simulink model "led_model"  (R2020a)
settings: Solver=FixedStepAuto  StartTime=0.0  StopTime=10.0  FixedStep=1e-3  RelTol=1e-3  EnableMultiTasking=on
undefined symbols (not defined in the file): D0, D1, D10, D11, D12, D13, D2, D3, D4, D5, D6, D7, D8, D9, PTA0, PTA1, PTA2, PTB23, PTB9, PTC16, PTC17, PTC2, PTC3, PTC4, PTD0, PTD1, PTD2, PTD3
libraries: frdmk64flib x17
settings Model: ExtModeTrigDuration=5  Creator=user  LastModifiedBy=user
settings OptimizationCC: EnhancedBackFolding=on  PassReuseOutputArgsAs=Individual arguments  ZeroExternalMemoryAtStartup=off  ZeroInternalMemoryAtStartup=off  MaxStackSize=64  OptimizeBlockOrder=speed  DifferentSizesBufferReuse=on  OptimizationCustomize=off  EfficientTunableParamExpr=on
settings DebuggingCC: ParameterTunabilityLossMsg=error
settings HardwareCC: ProdBitPerPointer=32  ProdBitPerSizeT=32  ProdBitPerPtrDiffT=32  ProdLargestAtomicInteger=Long  ProdLargestAtomicFloat=Double  ProdWordSize=32  ProdHWDeviceType=ARM Compatible->ARM Cortex
settings SFSimCC: MATLABDynamicMemAlloc=off
settings RTWCC: SystemTargetFile=ert.tlc  HardwareBoard=NXP FRDM-K64F  TemplateMakefile=ert_default_tmf  Toolchain=GNU Tools for ARM Embedded Processors
settings CodeAppCC: ForceParamTrailComments=on  IgnoreCustomStorageClasses=off  OperatorAnnotations=on  SimulinkDataObjDesc=on  SFDataObjDesc=on  InsertBlockDesc=on

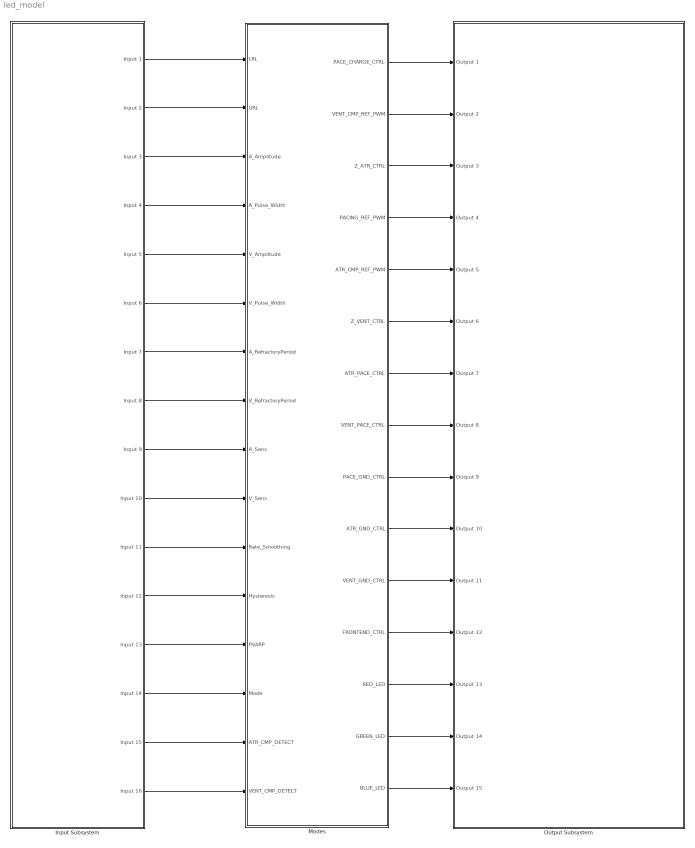
== system led_model ==
  Input Subsystem : Subsystem
  Modes : Stateflow chart  TreatAsAtomicUnit=on
  Output Subsystem : Subsystem
  wires:
  Modes/1(PACE_CHARGE_CTRL) -> Output Subsystem/1(Output 1)
  Modes/2(VENT_CMP_REF_PWM) -> Output Subsystem/2(Output 2)
  Modes/3(Z_ATR_CTRL) -> Output Subsystem/3(Output 3)
  Modes/4(PACING_REF_PWM) -> Output Subsystem/4(Output 4)
  Modes/5(ATR_CMP_REF_PWM) -> Output Subsystem/5(Output 5)
  Modes/6(Z_VENT_CTRL) -> Output Subsystem/6(Output 6)
  Modes/7(ATR_PACE_CTRL) -> Output Subsystem/7(Output 7)
  Modes/8(VENT_PACE_CTRL) -> Output Subsystem/8(Output 8)
  Modes/9(PACE_GND_CTRL) -> Output Subsystem/9(Output 9)
  Modes/10(ATR_GND_CTRL) -> Output Subsystem/10(Output 10)
  Modes/11(VENT_GND_CTRL) -> Output Subsystem/11(Output 11)
  Modes/12(FRONTEND_CTRL) -> Output Subsystem/12(Output 12)
  Modes/13(RED_LED) -> Output Subsystem/13(Output 13)
  Modes/14(GREEN_LED) -> Output Subsystem/14(Output 14)
  Modes/15(BLUE_LED) -> Output Subsystem/15(Output 15)
  Input Subsystem/1(Input 1) -> Modes/1(LRL)
  Input Subsystem/2(Input 2) -> Modes/2(URL)
  Input Subsystem/3(Input 3) -> Modes/3(A_Amplitude)
  Input Subsystem/4(Input 4) -> Modes/4(A_Pulse_Width)
  Input Subsystem/5(Input 5) -> Modes/5(V_Amplitude)
  Input Subsystem/6(Input 6) -> Modes/6(V_Pulse_Width)
  Input Subsystem/9(Input 9) -> Modes/9(A_Sens)
  Input Subsystem/10(Input 10) -> Modes/10(V_Sens)
  Input Subsystem/11(Input 11) -> Modes/11(Rate_Smoothing)
  Input Subsystem/12(Input 12) -> Modes/12(Hysteresis)
  Input Subsystem/13(Input 13) -> Modes/13(PVARP)
  Input Subsystem/14(Input 14) -> Modes/14(Mode)
  Input Subsystem/15(Input 15) -> Modes/15(ATR_CMP_DETECT)
  Input Subsystem/16(Input 16) -> Modes/16(VENT_CMP_DETECT)
  Input Subsystem/7(Input 7) -> Modes/7(A_RefractoryPeriod)
  Input Subsystem/8(Input 8) -> Modes/8(V_RefractoryPeriod)

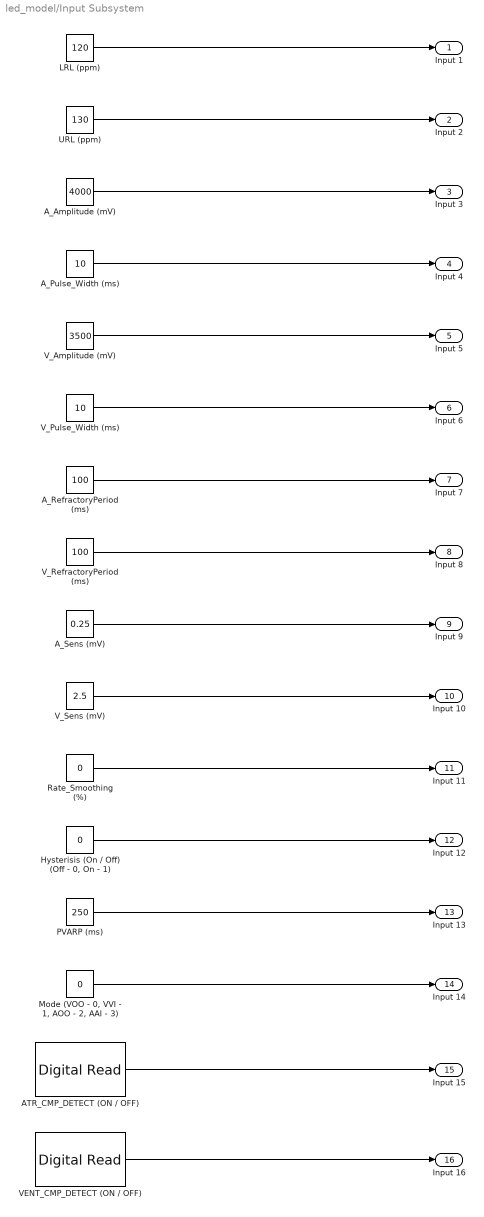
== system led_model/Input Subsystem ==
  ATR_CMP_DETECT (ON / OFF) : frdmk64flib/Digital Read  Whichpin=PTC16 (D0)  SampleTime=-1
  A_Amplitude (mV) : Constant  Value=4000
  A_Pulse_Width (ms) : Constant  Value=10
  A_RefractoryPeriod (ms) : Constant  Value=100
  A_Sens (mV) : Constant  Value=0.25
  "Hysterisis (On / Off) (Off - 0, On - 1)" : Constant  Value=0
  LRL (ppm) : Constant  Value=120
  "Mode (VOO - 0, VVI - 1, AOO - 2, AAI - 3)" : Constant  Value=0
  PVARP (ms) : Constant  Value=250
  Rate_Smoothing (%) : Constant  Value=0
  URL (ppm) : Constant  Value=130
  VENT_CMP_DETECT (ON / OFF) : frdmk64flib/Digital Read  Whichpin=PTC17 (D1)  SampleTime=-1
  V_Amplitude (mV) : Constant  Value=3500
  V_Pulse_Width (ms) : Constant  Value=10
  V_RefractoryPeriod (ms) : Constant  Value=100
  V_Sens (mV) : Constant  Value=2.5
  Input 1 : Outport
  Input 2 : Outport  Port=2
  Input 3 : Outport  Port=3
  Input 4 : Outport  Port=4
  Input 5 : Outport  Port=5
  Input 6 : Outport  Port=6
  Input 7 : Outport  Port=7
  Input 8 : Outport  Port=8
  Input 9 : Outport  Port=9
  Input 10 : Outport  Port=10
  Input 11 : Outport  Port=11
  Input 12 : Outport  Port=12
  Input 13 : Outport  Port=13
  Input 14 : Outport  Port=14
  Input 15 : Outport  Port=15
  Input 16 : Outport  Port=16
  wires:
  V_RefractoryPeriod (ms)/1 -> Input 8/1
  URL (ppm)/1 -> Input 2/1
  VENT_CMP_DETECT (ON / OFF)/1 -> Input 16/1
  V_Pulse_Width (ms)/1 -> Input 6/1
  "Mode (VOO - 0, VVI - 1, AOO - 2, AAI - 3)"/1 -> Input 14/1
  ATR_CMP_DETECT (ON / OFF)/1 -> Input 15/1
  A_Amplitude (mV)/1 -> Input 3/1
  V_Sens (mV)/1 -> Input 10/1
  A_Pulse_Width (ms)/1 -> Input 4/1
  PVARP (ms)/1 -> Input 13/1
  LRL (ppm)/1 -> Input 1/1
  A_Sens (mV)/1 -> Input 9/1
  V_Amplitude (mV)/1 -> Input 5/1
  A_RefractoryPeriod (ms)/1 -> Input 7/1
  Rate_Smoothing (%)/1 -> Input 11/1
  "Hysterisis (On / Off) (Off - 0, On - 1)"/1 -> Input 12/1

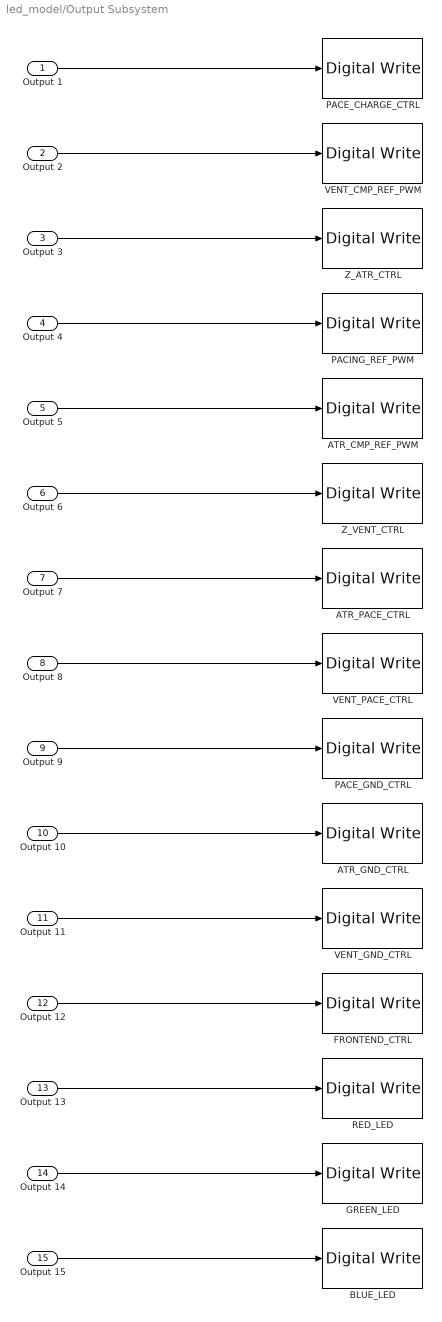
== system led_model/Output Subsystem ==
  Output 1 : Inport
  Output 2 : Inport  Port=2
  Output 3 : Inport  Port=3
  Output 4 : Inport  Port=4
  Output 5 : Inport  Port=5
  Output 6 : Inport  Port=6
  Output 7 : Inport  Port=7
  Output 8 : Inport  Port=8
  Output 9 : Inport  Port=9
  Output 10 : Inport  Port=10
  Output 11 : Inport  Port=11
  Output 12 : Inport  Port=12
  Output 13 : Inport  Port=13
  Output 14 : Inport  Port=14
  Output 15 : Inport  Port=15
  ATR_CMP_REF_PWM : frdmk64flib/Digital Write  Whichpin=PTC2 (D6)
  ATR_GND_CTRL : frdmk64flib/Digital Write  Whichpin=PTD2 (D11)
  ATR_PACE_CTRL : frdmk64flib/Digital Write  Whichpin=PTA0 (D8)
  BLUE_LED : frdmk64flib/Digital Write  Whichpin=BLUE_LED
  FRONTEND_CTRL : frdmk64flib/Digital Write  Whichpin=PTD1 (D13)
  GREEN_LED : frdmk64flib/Digital Write  Whichpin=GREEN_LED
  PACE_CHARGE_CTRL : frdmk64flib/Digital Write  Whichpin=PTB9 (D2)
  PACE_GND_CTRL : frdmk64flib/Digital Write  Whichpin=PTD0 (D10)
  PACING_REF_PWM : frdmk64flib/Digital Write  Whichpin=PTA2 (D5)
  RED_LED : frdmk64flib/Digital Write  Whichpin=RED_LED
  VENT_CMP_REF_PWM : frdmk64flib/Digital Write  Whichpin=PTA1 (D3)
  VENT_GND_CTRL : frdmk64flib/Digital Write  Whichpin=PTD3 (D12)
  VENT_PACE_CTRL : frdmk64flib/Digital Write  Whichpin=PTC4 (D9)
  Z_ATR_CTRL : frdmk64flib/Digital Write  Whichpin=PTB23 (D4)
  Z_VENT_CTRL : frdmk64flib/Digital Write  Whichpin=PTC3 (D7)
  wires:
  Output 11/1 -> VENT_GND_CTRL/1
  Output 1/1 -> PACE_CHARGE_CTRL/1
  Output 10/1 -> ATR_GND_CTRL/1
  Output 15/1 -> BLUE_LED/1
  Output 3/1 -> Z_ATR_CTRL/1
  Output 13/1 -> RED_LED/1
  Output 6/1 -> Z_VENT_CTRL/1
  Output 9/1 -> PACE_GND_CTRL/1
  Output 8/1 -> VENT_PACE_CTRL/1
  Output 4/1 -> PACING_REF_PWM/1
  Output 5/1 -> ATR_CMP_REF_PWM/1
  Output 7/1 -> ATR_PACE_CTRL/1
  Output 2/1 -> VENT_CMP_REF_PWM/1
  Output 12/1 -> FRONTEND_CTRL/1
  Output 14/1 -> GREEN_LED/1

== stateflow chart led_model/Modes ==
  note: Since in the main state, FRONTEND_CTRL is true so the
      | microcontroller enables sensing. The pacemaker then waits
      | until after the ventricle refractory period (V_RefractoryPeriod)
      | and if the current mode is set to VVI (Mode 1) and the
      | microcontroller senses a natural pace in the ventricle
      | (VENT_CMP_DETECT is true), it loops back into VOO_Charging
      | to inhibit the next ventricle pace. The microcontroller registers a
      | pace when the ventricle threshold sensitivity is exceeded which
      | is represented by the value of V_Sens stored into
      | VENT_CMP_REF_PWM. After using the MCP6546 Comparator
      | within the microcontroller to compare the rectified signal and
      | the PWM threshold, the output would trigger a response through
      | the VENT_CMP_DETECT pin which indicates that the ventricle
      | triggered a pulse.
  state VVI
    %To show when Ventricular pace being inhibited
    entry:
    RED_LED = true;
  state VOO_Pacing
    %Discharging C22
    entry:
    PACE_CHARGE_CTRL = false;
    PACE_GND_CTRL = true;
    ATR_PACE_CTRL = false;
    ATR_GND_CTRL = false;
    Z_ATR_CTRL = false;
    Z_VENT_CTRL = false;
    VENT_GND_CTRL = false;
    VENT_PACE_CTRL = true;
    GREEN_LED = true;
  state VOO_Charging
    %Charging C22 and Discharging Blocking Capacitor
    entry:
    ATR_PACE_CTRL = false;
    VENT_PACE_CTRL = false;
    PACING_REF_PWM = V_Amplitude;
    PACE_CHARGE_CTRL = true;
    %Discharging Blocking Capacitor
    PACE_GND_CTRL = true;
    Z_ATR_CTRL = false;
    Z_VENT_CTRL = false;
    ATR_GND_CTRL = false;
    VENT_GND_CTRL = true;
    GREEN_LED = false;
    %Needed for VENT_CMP_DETECT
    VENT_CMP_REF_PWM = V_Sens;
  note: The state becomes ready for pacing after a delay
      | which is indicated by the time interval between
      | the ventricle paces. This time interval is represented
      | by 60000 divided by the lower rate limit in ppm
      | subtracted by the programmed ventricular pulse width.
  note: If the mode is set to VOO or VVI,
      | proceed to the next state
  note: Move from ventricle pacing state back to charging
      | the C22 capacitor after the programmed ventricle
      | pulse width.
  note: In the charging state, the C22 capacitor is charged and the blocking
      | capacitor is discharged. To charge the C22 capacitor,
      | PACE_CHARGE_CTRL is set to true to charge the pacing capacitor,
      | and both ATR_PACE_CTRL and VENT_PACE_CTRL is set to false
      | to prevent the patient from being directly connected to the input
      | charging signal. To simultaneously discharge the blocking capacitor,
      | the net charge build-up in the ventricle/atrium must be reduced to
      | zero. For the specific mode, the GND_CTRL is set to true to act as
      | a pull-down for the electrode in order to prevent unwanted pacing.
      | The GND_CTRL for the other mode is set to false along with the
      | Z_ATR_CTRL and Z_VENT_CTRL so there is no impedance in the
      | respective chambers.
  note: In the pacing state, the charged C22 capacitor applies a pace to
      | either the ventricle or atirum depending on the mode. The power
      | supply is cut off the circuit by setting PACE_CHARGE_CTRL
      | to false and the switch PACE_CTRL is turned on to direct current
      | towards the specific chamber for the current mode. Only the specific
      | pacing switch for the current mode is true while the other is made
      | false to prevent parallel connection. The GND_CTRL for both atrial
      | and ventricular are turned false to ensure that the pacing signals
      | do not flow back into ground. Z_ATR_CTRL and Z_VENT_CTRL
      | remains false so that there is no impedance within the atrial and
      | ventricular chambers.
  state Main
    entry:
    BLUE_LED = false;
    RED_LED = false;
    GREEN_LED = false;
    PACING_REF_PWM = 0;
    FRONTEND_CTRL = true;
  note: In the main state, all LED indicators are
      | initialized to false. The variable
      | FRONTEND_CTRL is initialized to true in
      | order to activate sensing. There are two
      |  transitions to the other states based on
      | the mode that was selected.
  state AOO_Charging
    %Charging C22 and Discharging Blocking Capacitor
    entry:
    ATR_PACE_CTRL = false;
    VENT_PACE_CTRL = false;
    PACING_REF_PWM = A_Amplitude;
    PACE_CHARGE_CTRL = true;
    %Discharging Blocking Capacitor
    PACE_GND_CTRL = true;
    Z_ATR_CTRL = false;
    Z_VENT_CTRL = false;
    ATR_GND_CTRL = true;
    VENT_GND_CTRL = false;
    BLUE_LED=false;
    RED_LED = false;
    %Needed for ATR_CMP_DETECT
    ATR_CMP_REF_PWM = A_Sens;
  note: The state becomes ready for pacing after a delay
      | which is indicated by the time interval between
      | the atrial paces. This time interval is represented
      | by 60000 divided by the lower rate limit in ppm
      | subtracted by the programmed atrial pulse width.
  state AOO_Pacing
    %Discharging C22
    entry:
    PACE_CHARGE_CTRL = false;
    PACE_GND_CTRL = true;
    ATR_PACE_CTRL = true;
    ATR_GND_CTRL = false;
    Z_ATR_CTRL = false;
    Z_VENT_CTRL = false;
    VENT_GND_CTRL = false;
    VENT_PACE_CTRL = false;
    BLUE_LED = true;
  note: If the mode is set to AOO or AAI,
      | proceed to the next state
  note: Move from atrial pacing state back to charging
      | the C22 capacitor after the programmed atrial
      | pulse width.
  state AAI
    %To show when Atrial pace being inhibited
    entry:
    RED_LED = true;
  note: Since in the main state, FRONTEND_CTRL is true so the
      | microcontroller enables sensing. The pacemaker then waits
      | until after the atrial refractory period (A_RefractoryPeriod)
      | and if the current mode is set to AAI (Mode 3) and the
      | microcontroller senses a natural pace in the atrium
      | (ATR_CMP_DETECT is true), it loops back into AOO_Charging
      | to inhibit the next atrium pace. The microcontroller registers a
      | pace when the atrium threshold sensitivity is exceeded which
      | is represented by the value of A_Sens stored into
      | ATR_CMP_REF_PWM. After using the MCP6546 Comparator
      | within the microcontroller to compare the rectified signal and
      | the PWM threshold, the output would trigger a response through
      | the ATR_CMP_DETECT pin which indicates that the atrium triggered
      | a pulse.
  VOO_Charging -> VVI [order 2] : [after(V_RefractoryPeriod, msec) && Mode == 1 && VENT_CMP_DETECT == true]
  VVI -> VOO_Charging
  VOO_Charging -> VOO_Pacing [order 1] : after([60000/LRL] - V_Pulse_Width, msec)
  Main -> VOO_Charging [order 2] : [Mode == 0 || Mode == 1]
  VOO_Pacing -> VOO_Charging : after(V_Pulse_Width,msec)
  (default) -> Main
  Main -> AOO_Charging [order 1] : [Mode==2 || Mode == 3]
  AOO_Charging -> AOO_Pacing [order 1] : after([60000/LRL] - A_Pulse_Width, msec)
  AOO_Pacing -> AOO_Charging : after(A_Pulse_Width,msec)
  AOO_Charging -> AAI [order 2] : [after(A_RefractoryPeriod, msec) && Mode == 3 && ATR_CMP_DETECT == true]
  AAI -> AOO_Charging
  data: PACE_CHARGE_CTRL output; VENT_CMP_REF_PWM output; Z_ATR_CTRL output; PACING_REF_PWM output; ATR_CMP_REF_PWM output; Z_VENT_CTRL output; LRL input; URL input; A_Amplitude input; A_Pulse_Width input; ATR_PACE_CTRL output; VENT_PACE_CTRL output; PACE_GND_CTRL output; ATR_GND_CTRL output; VENT_GND_CTRL output; FRONTEND_CTRL output; V_Amplitude input; V_Pulse_Width input; A_RefractoryPeriod input; RED_LED output; GREEN_LED output; BLUE_LED output; V_RefractoryPeriod input; A_Sens input; V_Sens input; Rate_Smoothing input; Hysteresis input; PVARP input; Mode input; ATR_CMP_DETECT input; VENT_CMP_DETECT input
